simulink model "actividad_clase_control"  (R2024a)
settings: Solver=VariableStepAuto  StartTime=0.0  StopTime=400  RelTol=1e-3
undefined symbols (not defined in the file): denTF, KD, KI, KP, numTF
libraries: fuzblock x1
settings Model: Creator=srsue  LastModifiedBy=srsue

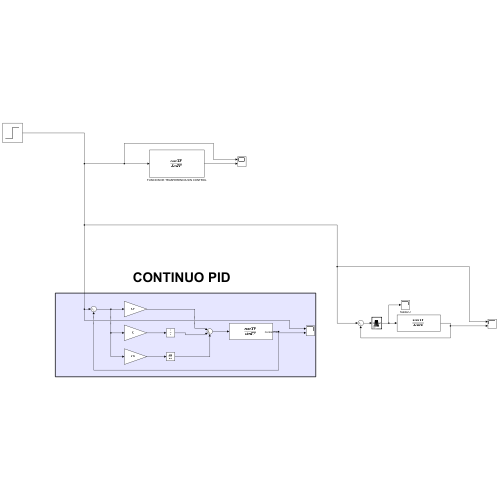
[thumbnail: Simulink's stored preview of the top-level diagram]
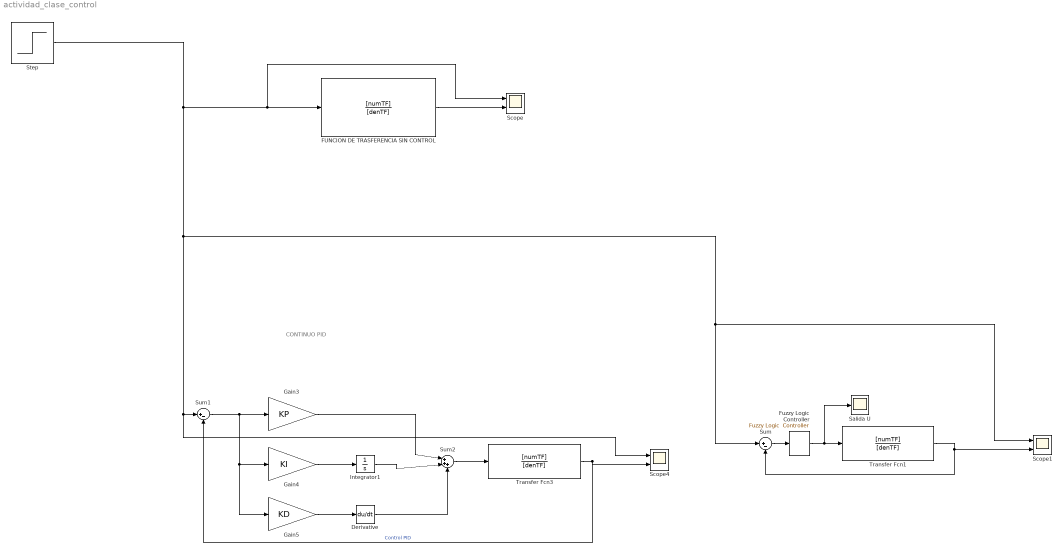
== system actividad_clase_control ==
  note: CONTINUO PID
  Derivative : Derivative
  FUNCION DE TRASFERENCIA SIN CONTROL : TransferFcn  Numerator=[numTF]  Denominator=[denTF]
  Fuzzy Logic Controller : fuzblock/Fuzzy Logic  Controller  FIS=control_temperatura  OutputSampleNumber=101  DataType=double  FuzzifiedInputs=off  RuleFiringStrengths=off  RuleOutputs=off  AggregatedOutputs=off  SimulateUsing=Interpreted execution  OutOfRangeInputValueMessage=warning  NoRuleFiredMessage=warning  EmptyOutputFuzzySetMessage=warning
  Gain3 : Gain  Gain=KP
  Gain4 : Gain  Gain=KI
  Gain5 : Gain  Gain=KD
  Integrator1 : Integrator
  Salida U : Scope
  Scope : Scope  NumInputPorts=2
  Scope1 : Scope  NumInputPorts=2
  Scope4 : Scope  NumInputPorts=2
  Step : Step  After=80  SampleTime=0
  Sum : Sum  Inputs=|+-
  Sum1 : Sum  Inputs=|+-
  Sum2 : Sum  Inputs=|+++
  Transfer Fcn1 : TransferFcn  Numerator=[numTF]  Denominator=[denTF]
  Transfer Fcn3 : TransferFcn  Numerator=[numTF]  Denominator=[denTF]
  wires:
  Sum1/1 -> Gain5/1, Gain4/1, Gain3/1
  Gain3/1 -> Sum2/1
  Derivative/1 -> Sum2/3
  Gain5/1 -> Derivative/1
  Transfer Fcn3/1 -> Scope4/2, Sum1/2  "Control PID"
  Gain4/1 -> Integrator1/1
  Sum2/1 -> Transfer Fcn3/1
  Integrator1/1 -> Sum2/2
  FUNCION DE TRASFERENCIA SIN CONTROL/1 -> Scope/2
  Fuzzy Logic Controller/1 -> Transfer Fcn1/1, Salida U/1
  Step/1 -> Scope/1, FUNCION DE TRASFERENCIA SIN CONTROL/1, Scope1/1, Sum/1, Sum1/1, Scope4/1
  Transfer Fcn1/1 -> Sum/2, Scope1/2
  Sum/1 -> Fuzzy Logic Controller/1
